simulink model "AME556_Project_Task5_v4"  (R2024b)
settings: Solver=daessc  StartTime=0.0  StopTime=10  FixedStep=0.0005  MaxStep=1e-3  RelTol=1e-2
InitFcn:
  | global params;
  | 
  | % Mass and geometry
  | params.m = 0.25;
  | params.l = 0.22;
  | params.mb = 8;
  | params.a = 0.25;
  | params.b = 0.15;
  | params.g = [0; 9.81; 0];
  | 
  | % Moment of inerita
  | Il_zz = params.m * params.l^2 / 12;
  | Ib_xx = params.mb * params.a^2 / 12;
  | Ib_yy = params.mb * params.b^2 / 12;
  | Ib_zz = params.mb * (params.a^2 + params.b^2) / 12;
  | params.Ib = diag([Ib_xx Ib_yy Ib_zz]);
  | 
  | % Spatial contact force parameters
  | Kp_g = 1e5;
  | Kd_g = 1e3;
  | 
  | % Ground contact positions
  | params.P1 = [0.0197; 0.0022; 0];
  | params.P2 = [0.1838; 0.0041; 0];
  | 
  | % State variables
  | q0 = [0.1; 0.45; 0; -pi/3; pi/2; -pi/6; pi/2]; % Initial states (before landing)
  | params.p_d = [0; 0.5; 0]; % Desired positions (after standing): [x_d; y_d; z_d];
  | params.theta_d = 0; % Desired angle
values from neighbouring files (symbols this model uses):
  dt = 0.04    [AME556_Project_Task5_Setup.m]
  l = 0.5    [AME556_Project_Task5_Setup.m]
  N = 10    [AME556_Project_Task5_Setup.m]
undefined symbols (not defined in the file or in its folder): P1_world0, P2_world0, X, Y, Z
libraries: sm_lib x29, nesl_utility x27
(part 2 of 2)

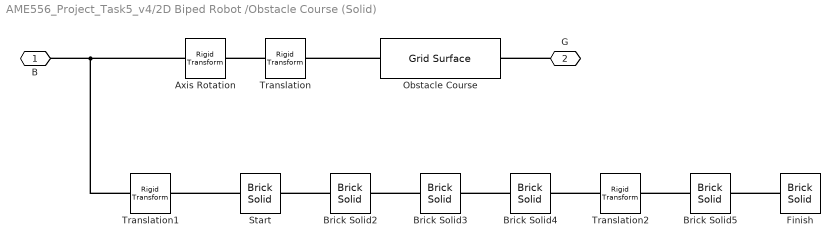
== system AME556_Project_Task5_v4/2D Biped Robot /Obstacle Course (Solid) ==
  Axis Rotation : sm_lib/Frames and Transforms/Rigid Transform  RotationMethod=AlignedAxes  FollAlignAxisA=+X  BaseAlignAxisA=+Z  FollAlignAxisB=+Y  BaseAlignAxisB=+X  RotationStandardAxis=+Z  RotationAngle=0  RotationAngleUnits=deg  RotationArbitraryAxis=[0 0 1]  RotationSequenceAxes=FollowerAxes  RotationSequence=XYX  RotationSequenceAngles=[0 0 0]  RotationSequenceAnglesUnits=deg  RotationMatrix=[1 0 0;0 1 0;0 0 1]  Quaternion=[1 0 0 0]  TranslationMethod=StandardAxis  TranslationCartesianOffset=[0 0 0]  TranslationCartesianOffsetUnits=m  TranslationStandardAxis=-Z  TranslationStandardOffset=0.5  TranslationStandardOffsetUnits=m  TranslationROffset=0  TranslationROffsetUnits=m  TranslationThetaOffset=0  TranslationThetaOffsetUnits=deg  TranslationZOffset=0  TranslationZOffsetUnits=m
  Brick Solid2 : sm_lib/Body Elements/Brick Solid  BrickDimensions=[2 0.4 1]  BrickDimensionsUnits=m  ExportEntireGeometry=off  InertiaType=CalculateFromGeometry  BasedOnType=Density  Density=1000  DensityUnits=kg/m^3  Mass=1  MassUnits=kg  CenterOfMass=[0 0 0]  CenterOfMassUnits=m  MomentsOfInertia=[1 1 1]  MomentsOfInertiaUnits=kg*m^2  ProductsOfInertia=[0 0 0]  ProductsOfInertiaUnits=kg*m^2  GraphicType=FromGeometry  MarkerShape=Sphere  MarkerSize=10  GraphicVisPropType=SimpleVisualProperties  GraphicDiffuseColor=[0.5 0.5 0.5]  GraphicOpacity=1  GraphicSpecularColor=[0.5 0.5 0.5 1.0]  GraphicAmbientColor=[0.15 0.15 0.15 1.0]  GraphicEmissiveColor=[0.0 0.0 0.0 1.0]  GraphicShininess=75  DoExposeReferenceFrame=off  SerializedFrames=<Frames><Frame><Id>Frame1</Id><Value><Name>F1</Name><Origin><Source>GeometricFeature</Source><FeatureName>-x +y curve</FeatureName></Origin><PrimaryAxis><DefinedDirection>+Z</DefinedDirection><Source>ReferenceFrame</Source><SourceDirection>+Z</SourceDirection><FeatureName></FeatureName></PrimaryAxis><SecondaryAxis><DefinedDirection>+X</DefinedDirection><Source>ReferenceFrame</Source><SourceDirection>+X</SourceDirection><FeatureName></FeatureName></SecondaryAxis></Value></Frame><Frame><Id>Frame2</Id><Value><Name>F2</Name><Origin><Source>GeometricFeature</Source><FeatureName>+x -y curve</FeatureName></Origin><PrimaryAxis><DefinedDirection>+Z</DefinedDirection><Source>ReferenceFrame</Source><SourceDirection>+Z</SourceDirection><FeatureName></FeatureName></PrimaryAxis><SecondaryAxis><DefinedDirection>+X</DefinedDirection><Source>ReferenceFrame</Source><SourceDirection>+X</SourceDirection><FeatureName></FeatureName></SecondaryAxis></Value></Frame></Frames>
  Brick Solid3 : sm_lib/Body Elements/Brick Solid  BrickDimensions=[1 0.8 1]  BrickDimensionsUnits=m  ExportEntireGeometry=off  InertiaType=CalculateFromGeometry  BasedOnType=Density  Density=1000  DensityUnits=kg/m^3  Mass=1  MassUnits=kg  CenterOfMass=[0 0 0]  CenterOfMassUnits=m  MomentsOfInertia=[1 1 1]  MomentsOfInertiaUnits=kg*m^2  ProductsOfInertia=[0 0 0]  ProductsOfInertiaUnits=kg*m^2  GraphicType=FromGeometry  MarkerShape=Sphere  MarkerSize=10  GraphicVisPropType=SimpleVisualProperties  GraphicDiffuseColor=[0.5 0.5 0.5]  GraphicOpacity=1  GraphicSpecularColor=[0.5 0.5 0.5 1.0]  GraphicAmbientColor=[0.15 0.15 0.15 1.0]  GraphicEmissiveColor=[0.0 0.0 0.0 1.0]  GraphicShininess=75  DoExposeReferenceFrame=off  SerializedFrames=<Frames><Frame><Id>Frame1</Id><Value><Name>F1</Name><Origin><Source>GeometricFeature</Source><FeatureName>-x -y curve</FeatureName></Origin><PrimaryAxis><DefinedDirection>+Z</DefinedDirection><Source>ReferenceFrame</Source><SourceDirection>+Z</SourceDirection><FeatureName></FeatureName></PrimaryAxis><SecondaryAxis><DefinedDirection>+X</DefinedDirection><Source>ReferenceFrame</Source><SourceDirection>+X</SourceDirection><FeatureName></FeatureName></SecondaryAxis></Value></Frame><Frame><Id>Frame2</Id><Value><Name>F2</Name><Origin><Source>GeometricFeature</Source><FeatureName>+x -y curve</FeatureName></Origin><PrimaryAxis><DefinedDirection>+Z</DefinedDirection><Source>ReferenceFrame</Source><SourceDirection>+Z</SourceDirection><FeatureName></FeatureName></PrimaryAxis><SecondaryAxis><DefinedDirection>+X</DefinedDirection><Source>ReferenceFrame</Source><SourceDirection>+X</SourceDirection><FeatureName></FeatureName></SecondaryAxis></Value></Frame></Frames>
  Brick Solid4 : sm_lib/Body Elements/Brick Solid  BrickDimensions=[2 0.4 1]  BrickDimensionsUnits=m  ExportEntireGeometry=off  InertiaType=CalculateFromGeometry  BasedOnType=Density  Density=1000  DensityUnits=kg/m^3  Mass=1  MassUnits=kg  CenterOfMass=[0 0 0]  CenterOfMassUnits=m  MomentsOfInertia=[1 1 1]  MomentsOfInertiaUnits=kg*m^2  ProductsOfInertia=[0 0 0]  ProductsOfInertiaUnits=kg*m^2  GraphicType=FromGeometry  MarkerShape=Sphere  MarkerSize=10  GraphicVisPropType=SimpleVisualProperties  GraphicDiffuseColor=[0.5 0.5 0.5]  GraphicOpacity=1  GraphicSpecularColor=[0.5 0.5 0.5 1.0]  GraphicAmbientColor=[0.15 0.15 0.15 1.0]  GraphicEmissiveColor=[0.0 0.0 0.0 1.0]  GraphicShininess=75  DoExposeReferenceFrame=off  SerializedFrames=<Frames><Frame><Id>Frame1</Id><Value><Name>F1</Name><Origin><Source>GeometricFeature</Source><FeatureName>-x -y curve</FeatureName></Origin><PrimaryAxis><DefinedDirection>+Z</DefinedDirection><Source>ReferenceFrame</Source><SourceDirection>+Z</SourceDirection><FeatureName></FeatureName></PrimaryAxis><SecondaryAxis><DefinedDirection>+X</DefinedDirection><Source>ReferenceFrame</Source><SourceDirection>+X</SourceDirection><FeatureName></FeatureName></SecondaryAxis></Value></Frame><Frame><Id>Frame2</Id><Value><Name>F2</Name><Origin><Source>GeometricFeature</Source><FeatureName>+x +y curve</FeatureName></Origin><PrimaryAxis><DefinedDirection>+Z</DefinedDirection><Source>ReferenceFrame</Source><SourceDirection>+Z</SourceDirection><FeatureName></FeatureName></PrimaryAxis><SecondaryAxis><DefinedDirection>+X</DefinedDirection><Source>ReferenceFrame</Source><SourceDirection>+X</SourceDirection><FeatureName></FeatureName></SecondaryAxis></Value></Frame></Frames>
  Brick Solid5 : sm_lib/Body Elements/Brick Solid  BrickDimensions=[2 0.4 1]  BrickDimensionsUnits=m  ExportEntireGeometry=off  InertiaType=CalculateFromGeometry  BasedOnType=Density  Density=1000  DensityUnits=kg/m^3  Mass=1  MassUnits=kg  CenterOfMass=[0 0 0]  CenterOfMassUnits=m  MomentsOfInertia=[1 1 1]  MomentsOfInertiaUnits=kg*m^2  ProductsOfInertia=[0 0 0]  ProductsOfInertiaUnits=kg*m^2  GraphicType=FromGeometry  MarkerShape=Sphere  MarkerSize=10  GraphicVisPropType=SimpleVisualProperties  GraphicDiffuseColor=[0.5 0.5 0.5]  GraphicOpacity=1  GraphicSpecularColor=[0.5 0.5 0.5 1.0]  GraphicAmbientColor=[0.15 0.15 0.15 1.0]  GraphicEmissiveColor=[0.0 0.0 0.0 1.0]  GraphicShininess=75  DoExposeReferenceFrame=off  SerializedFrames=<Frames><Frame><Id>Frame1</Id><Value><Name>F1</Name><Origin><Source>GeometricFeature</Source><FeatureName>-x +y curve</FeatureName></Origin><PrimaryAxis><DefinedDirection>+Z</DefinedDirection><Source>ReferenceFrame</Source><SourceDirection>+Z</SourceDirection><FeatureName></FeatureName></PrimaryAxis><SecondaryAxis><DefinedDirection>+X</DefinedDirection><Source>ReferenceFrame</Source><SourceDirection>+X</SourceDirection><FeatureName></FeatureName></SecondaryAxis></Value></Frame><Frame><Id>Frame2</Id><Value><Name>F2</Name><Origin><Source>GeometricFeature</Source><FeatureName>+x +y curve</FeatureName></Origin><PrimaryAxis><DefinedDirection>+Z</DefinedDirection><Source>ReferenceFrame</Source><SourceDirection>+Z</SourceDirection><FeatureName></FeatureName></PrimaryAxis><SecondaryAxis><DefinedDirection>+X</DefinedDirection><Source>ReferenceFrame</Source><SourceDirection>+X</SourceDirection><FeatureName></FeatureName></SecondaryAxis></Value></Frame></Frames>
  Finish : sm_lib/Body Elements/Brick Solid  BrickDimensions=[l 0.4 1]  BrickDimensionsUnits=m  ExportEntireGeometry=off  InertiaType=CalculateFromGeometry  BasedOnType=Density  Density=1000  DensityUnits=kg/m^3  Mass=1  MassUnits=kg  CenterOfMass=[0 0 0]  CenterOfMassUnits=m  MomentsOfInertia=[1 1 1]  MomentsOfInertiaUnits=kg*m^2  ProductsOfInertia=[0 0 0]  ProductsOfInertiaUnits=kg*m^2  GraphicType=FromGeometry  MarkerShape=Sphere  MarkerSize=10  GraphicVisPropType=SimpleVisualProperties  GraphicDiffuseColor=[0 1 0]  GraphicOpacity=1  GraphicSpecularColor=[0.5 0.5 0.5 1.0]  GraphicAmbientColor=[0.15 0.15 0.15 1.0]  GraphicEmissiveColor=[0.0 0.0 0.0 1.0]  GraphicShininess=75  DoExposeReferenceFrame=off  SerializedFrames=<Frames><Frame><Id>Frame1</Id><Value><Name>F1</Name><Origin><Source>GeometricFeature</Source><FeatureName>-x +y curve</FeatureName></Origin><PrimaryAxis><DefinedDirection>+Z</DefinedDirection><Source>ReferenceFrame</Source><SourceDirection>+Z</SourceDirection><FeatureName></FeatureName></PrimaryAxis><SecondaryAxis><DefinedDirection>+X</DefinedDirection><Source>ReferenceFrame</Source><SourceDirection>+X</SourceDirection><FeatureName></FeatureName></SecondaryAxis></Value></Frame></Frames>
  Obstacle Course : sm_lib/Curves and Surfaces/Grid Surface  XGridVector=x_grid  XGridVectorUnits=m  YGridVector=y_grid  YGridVectorUnits=m  ZHeights=z_height  ZHeightsUnits=m  GraphicType=FromGeometry  GraphicVisPropType=SimpleVisualProperties  GraphicDiffuseColor=[1 1 1]  GraphicOpacity=1  GraphicSpecularColor=[0.5 0.5 0.5 1.0]  GraphicAmbientColor=[0.15 0.15 0.15 1.0]  GraphicEmissiveColor=[0.0 0.0 0.0 1.0]  GraphicShininess=75
  Start : sm_lib/Body Elements/Brick Solid  BrickDimensions=[l 0.4 1]  BrickDimensionsUnits=m  ExportEntireGeometry=off  InertiaType=CalculateFromGeometry  BasedOnType=Density  Density=1000  DensityUnits=kg/m^3  Mass=1  MassUnits=kg  CenterOfMass=[0 0 0]  CenterOfMassUnits=m  MomentsOfInertia=[1 1 1]  MomentsOfInertiaUnits=kg*m^2  ProductsOfInertia=[0 0 0]  ProductsOfInertiaUnits=kg*m^2  GraphicType=FromGeometry  MarkerShape=Sphere  MarkerSize=10  GraphicVisPropType=SimpleVisualProperties  GraphicDiffuseColor=[1 0 0]  GraphicOpacity=1  GraphicSpecularColor=[0.5 0.5 0.5 1.0]  GraphicAmbientColor=[0.15 0.15 0.15 1.0]  GraphicEmissiveColor=[0.0 0.0 0.0 1.0]  GraphicShininess=75  DoExposeReferenceFrame=off  SerializedFrames=<Frames><Frame><Id>Frame1</Id><Value><Name>F1</Name><Origin><Source>GeometricFeature</Source><FeatureName>-x +y curve</FeatureName></Origin><PrimaryAxis><DefinedDirection>+Z</DefinedDirection><Source>ReferenceFrame</Source><SourceDirection>+Z</SourceDirection><FeatureName></FeatureName></PrimaryAxis><SecondaryAxis><DefinedDirection>+X</DefinedDirection><Source>ReferenceFrame</Source><SourceDirection>+X</SourceDirection><FeatureName></FeatureName></SecondaryAxis></Value></Frame><Frame><Id>Frame2</Id><Value><Name>F2</Name><Origin><Source>GeometricFeature</Source><FeatureName>+x +y curve</FeatureName></Origin><PrimaryAxis><DefinedDirection>+Z</DefinedDirection><Source>ReferenceFrame</Source><SourceDirection>+Z</SourceDirection><FeatureName></FeatureName></PrimaryAxis><SecondaryAxis><DefinedDirection>+X</DefinedDirection><Source>ReferenceFrame</Source><SourceDirection>+X</SourceDirection><FeatureName></FeatureName></SecondaryAxis></Value></Frame></Frames>
  Translation : sm_lib/Frames and Transforms/Rigid Transform  RotationMethod=None  FollAlignAxisA=+X  BaseAlignAxisA=+Z  FollAlignAxisB=+Y  BaseAlignAxisB=+X  RotationStandardAxis=+Z  RotationAngle=0  RotationAngleUnits=deg  RotationArbitraryAxis=[0 0 1]  RotationSequenceAxes=FollowerAxes  RotationSequence=XYX  RotationSequenceAngles=[0 0 0]  RotationSequenceAnglesUnits=deg  RotationMatrix=[1 0 0;0 1 0;0 0 1]  Quaternion=[1 0 0 0]  TranslationMethod=StandardAxis  TranslationCartesianOffset=[0 0 0]  TranslationCartesianOffsetUnits=m  TranslationStandardAxis=-Y  TranslationStandardOffset=l  TranslationStandardOffsetUnits=m  TranslationROffset=0  TranslationROffsetUnits=m  TranslationThetaOffset=0  TranslationThetaOffsetUnits=deg  TranslationZOffset=0  TranslationZOffsetUnits=m
  Translation1 : sm_lib/Frames and Transforms/Rigid Transform  RotationMethod=None  FollAlignAxisA=+X  BaseAlignAxisA=+Z  FollAlignAxisB=+Y  BaseAlignAxisB=+X  RotationStandardAxis=+Z  RotationAngle=0  RotationAngleUnits=deg  RotationArbitraryAxis=[0 0 1]  RotationSequenceAxes=FollowerAxes  RotationSequence=XYX  RotationSequenceAngles=[0 0 0]  RotationSequenceAnglesUnits=deg  RotationMatrix=[1 0 0;0 1 0;0 0 1]  Quaternion=[1 0 0 0]  TranslationMethod=StandardAxis  TranslationCartesianOffset=[0 0 0]  TranslationCartesianOffsetUnits=m  TranslationStandardAxis=-X  TranslationStandardOffset=l  TranslationStandardOffsetUnits=m  TranslationROffset=0  TranslationROffsetUnits=m  TranslationThetaOffset=0  TranslationThetaOffsetUnits=deg  TranslationZOffset=0  TranslationZOffsetUnits=m
  Translation2 : sm_lib/Frames and Transforms/Rigid Transform  RotationMethod=None  FollAlignAxisA=+X  BaseAlignAxisA=+Z  FollAlignAxisB=+Y  BaseAlignAxisB=+X  RotationStandardAxis=+Z  RotationAngle=0  RotationAngleUnits=deg  RotationArbitraryAxis=[0 0 1]  RotationSequenceAxes=FollowerAxes  RotationSequence=XYX  RotationSequenceAngles=[0 0 0]  RotationSequenceAnglesUnits=deg  RotationMatrix=[1 0 0;0 1 0;0 0 1]  Quaternion=[1 0 0 0]  TranslationMethod=StandardAxis  TranslationCartesianOffset=[0 0 0]  TranslationCartesianOffsetUnits=m  TranslationStandardAxis=+X  TranslationStandardOffset=0.4  TranslationStandardOffsetUnits=m  TranslationROffset=0  TranslationROffsetUnits=m  TranslationThetaOffset=0  TranslationThetaOffsetUnits=deg  TranslationZOffset=0  TranslationZOffsetUnits=m
  Β : PMIOPort  Side=Left
  G : PMIOPort  Port=2  Side=Right
  connections:
  Translation1/LConn1 -- Β/RConn1 -- Axis Rotation/LConn1
  Brick Solid4/LConn1 -- Brick Solid3/RConn1
  Brick Solid2/LConn1 -- Start/RConn1
  Translation2/LConn1 -- Brick Solid4/RConn1
  Finish/LConn1 -- Brick Solid5/RConn1
  Brick Solid5/LConn1 -- Translation2/RConn1
  Brick Solid3/LConn1 -- Brick Solid2/RConn1
  Start/LConn1 -- Translation1/RConn1
  Obstacle Course/LConn1 -- Translation/RConn1
  Translation/LConn1 -- Axis Rotation/RConn1
  G/RConn1 -- Obstacle Course/RConn1

== matlab function AME556_Project_Task5_v4/MATLAB Function ==
  data: tau_unsaturated input; tau_saturated output; saturateSwitch input
function tau_saturated = tau_saturation(tau_unsaturated, saturateSwitch)
    if saturateSwitch == 1
        tau_limits = [30, 60, 30, 60];
    
        tau_saturated = tau_unsaturated;
    
        for i = 1:length(tau_unsaturated)
            if tau_unsaturated(i) > tau_limits(i)
                tau_saturated(i) = tau_limits(i);
                warning('Tau %d (%.2f) is saturated to %d', i, tau_unsaturated(i), tau_limits(i));
            elseif tau_unsaturated(i) < -tau_limits(i)
                tau_saturated(i) = -tau_limits(i);
                warning('Tau %d (%.2f) is saturated to -%d', i, tau_unsaturated(i), tau_limits(i));
            end
        end
    else
        tau_saturated = tau_unsaturated;
    end
end

== matlab function AME556_Project_Task5_v4/Controller/Condensed MPC Controller ==
  settings: updateMethod=DISCRETE
  data: p input; theta input; dp input; dtheta input; qs input; tau output; P1 input; P2 input; dP1 input; dP2 input; N input; dt input; t input
%% Function: Low Level Control

function tau = lowLevelControl(p, theta, dp, dtheta, qs, P1, P2, dP1, dP2, N, dt, t)

% 正常情况下我们就正常摆腿
if p(1)<=1.7
    gaitType = "walk"; % Walk from start

elseif p(1)>1.7 && p(1)<=2.1
    gaitType = "hop_stand"; % Ready to jump

    if P1(2)>0.05 && P2(2)>0.05 % Flight
        gaitType = "hop_flight"; 
    end
    
elseif p(1)>2.1 && p(1)<=3
    gaitType = "walk_on_obstacle"; % Walk on higher ground

elseif p(1)>3 && p(1)<=4
    gaitType = "walk"; % 

elseif p(1)>4 && p(1)<=4.9
    gaitType = "walk2"; % 回到平地走

elseif p(1)>4.9 && p(1)<=5.4
    gaitType = "gap"; 
    
    if P1(1)>5.4
        gaitType = "stand"; 
    end
    if P2(1)>5.0
        gaitType = "stand2";
    end

else
    gaitType = "walk2";
end

% disp(gaitType)

con = gaitSchedule(N, dt, t, gaitType);
F = condensed_mpc_controller(p, theta, dp, dtheta, P1, P2, N, dt, t, con, gaitType);
J = jacobianFcn(theta, qs);

tau = zeros(4, 1);
if con(1, 1) && con(2, 1)
    tau = -J' * F;
elseif con(1, 1) && ~con(2, 1)
    F_swing = swingLegControl(p, dp, P2, dP2, N, dt, t, gaitType);
    F_new = [F(1: 2); -F_swing];
    tau = -J' * F_new;
elseif con(2, 1) && ~con(1, 1)
    F_swing = swingLegControl(p, dp, P1, dP1, N, dt, t, gaitType);
    F_new = [-F_swing; F(3: 4)];
    tau = -J' * F_new;
else
    F_swing1 = swingLegControl(p, dp, P1, dP1, N, dt, t, gaitType);
    F_swing2 = swingLegControl(p, dp, P2, dP2, N, dt, t, gaitType);
    F_new = [-F_swing1; -F_swing2];
    tau = -J' * F_new;    
end

end

%% Function: Condensed MPC Controller

function F = condensed_mpc_controller(p, theta, dp, dtheta, P1, P2, N, dt, t, con, gaitType)

% Parameters
mt = 8;
a = 0.25;
b = 0.15;
g = [0; 9.81; 0];
Ib_zz = mt * (a^2 + b^2) / 12;

numStates = 7;
numCtrls = 4;
Q = diag([200 200 800 30 10 10 0]);
R = 0.0001*eye(numCtrls);

% q = [x; y; z; R1; dx; dy; dz; wbx; wby; wbz];
% X = [x; y; theta; dx; dy; dtheta; g];
X = zeros(numStates, 1);
X(1: 2) = p;
X(3) = theta;
X(4: 5) = dp;
X(6) = dtheta;
X(7) = g(2);

% Desired states
switch gaitType
    case "walk"
        X_d = [0.5*t; 0.40; 0; 0.5; 0; 0; g(2)];

    case "jump_up"
        X_d = [0.5*t; 0.80; 0; dp(1); 3; 0; g(2)]; 

    case "fly_up"
        % fly的时候其实都是F_swing，不计算mpc，直接return
        F = zeros(4,1);
        return;

    case "walk_on_obstacle"
        X_d = [p(1); 0.80; 0; 0; 0; 0; g(2)];
    
    case "walk2"
        X_d = [0.8*t; 0.40; 0; 0.8; 0; 0; g(2)];

    case "gap"
        X_d = [5.40; 0.40; 0; dp(1); 0; 0; g(2)];

    case "stand"
        X_d = [5.40; 0.40; 0; dp(1); 0; 0; g(2)];
    case "stand2"
        X_d = [5.40; 0.40; 0; dp(1); 0; 0; g(2)];       

    otherwise
        error("unknown gait type");
end


% Reference Trajectory
X_ref = getReferenceTrajectory(dt, N, p, theta, dp, dtheta, X_d);
y = reshape(X_ref, [numStates*N 1]);

r1 = P1 - p;
r2 = P2 - p;

% Linearized system (A, B)
A = [zeros(3)   eye(3)    zeros(3,1);
     zeros(3, numStates-1) [0; -1; 0];
     zeros(1, numStates)];

B = [zeros(3, numCtrls);
     eye(2)/mt eye(2)/mt;
     -r1(2)/Ib_zz r1(1)/Ib_zz -r2(2)/Ib_zz r2(1)/Ib_zz;
     zeros(1, numCtrls)];

% Discrete-time system matrices (Ak, Bk)
Ak = A * dt + eye(size(A, 1));
Bk = B * dt;

% Aqp
Aqp = [];
for i = 1: N
    Aqp = [Aqp; mpower(Ak, i)];
end

% bqp
Bqp = repmat(zeros(size(Bk)), N, N);
for i = 0: N-1
    element = mpower(Ak, i) * Bk;
    Bqp = Bqp + kron(diag(ones(1, N - i), -i), element);
end

% Condensation
L = kron(eye(N), Q);
K = kron(eye(N), R);

% Optimization weights (H, f)
H = 2*(Bqp'*L*Bqp + K);
f = 2*Bqp'*L*(Aqp*X - y);

% Inequality constraints (A_ineq, b_ineq)
Aineq_mu = kron(eye(2), [1 -0.7; -1 -0.7]);
Aineq_mu_N = kron(eye(N), Aineq_mu);
Aineq_F = kron(eye(2), [0 1; 0 -1]);
Aineq_F_N = kron(eye(N), Aineq_F);
Aineq = [Aineq_mu_N; Aineq_F_N];

bineq_mu = repmat([0; 0; 0; 0], N, 1);
bineq_f = [];
for i = 1: N
    bineq_f = [bineq_f; [250; -10]*con(1, i); [250; -10]*con(2, i)];
end
bineq = [bineq_mu; bineq_f];

% Initial guess
u0 = zeros(length(f), 1);

% Quadratic programming
options = optimoptions('quadprog', 'Algorithm', 'active-set', 'Display', 'off');
u_mpc = quadprog(H, f, Aineq, bineq, [], [], [], [], u0, options);

% Force inputs
F = u_mpc(1: numCtrls);

end


%% Function: Get Reference Geometry

function X_ref = getReferenceTrajectory(dt, N, p, theta, dp, dtheta, X_d)

X = [p; theta; dp; dtheta; 9.81];
X_ref = repmat(X, 1, N);

for i = 1: 3
    for k = 2: N
        if X_d(i + 3) ~= 0
            X_ref(i, k) = X(i) + X_d(i+3)*((k-1)*dt);
        else
            X_ref(i, k) = X_d(i);
        end
    end
end

end

%% Function: Swing Leg Control

function F_swing = swingLegControl(p, dp, P, dP, N, dt, t, gaitType)

Kp = diag([200 300]);
Kd = eye(2)*5;

del_t = N*dt/2;
ts = rem(t, del_t);

switch gaitType
    case "walk"
        % 正常摆腿逻辑
        swingHeight = 0.1; % 正常摆腿高度
        Px_d = p(1) + (1/2)*del_t*dp(1);
        Py_d = swingHeight * sin(pi*ts/del_t);
    
    case "hop_stand"
        % jump的时候其实双脚落地不会有F_swing，不计算F_swing，直接返回
        F_swing = zeros(2,1);
        return;

    case "hop_fligt"
        % 试图抬高双脚
        swingHeight = 0.2;
        Px_d = p(1) + (1/2)*del_t*dp(1);
        %Py_d = (1/2)*del_t*dp(2) + 2*(sin(pi*ts/del_t))^(1/3)*swingHeight;
        Py_d = 0.5;

    case "walk_on_obstacle"
        % 正常摆腿逻辑
        swingHeight = 0.1; % 正常摆腿高度
        Px_d = p(1) + (1/2)*del_t*dp(1);
        Py_d = (swingHeight+0.4) * sin(pi*ts/del_t);

    case "walk2"
        % 正常摆腿逻辑
        swingHeight = 0.1; % 正常摆腿高度
        Px_d = p(1) + (1/2)*del_t*dp(1);
        Py_d = swingHeight * sin(pi*ts/del_t);

    case "gap"
        % 试图单腿迈过沟
        swingHeight = 0.1; 
        Px_d = 5.8;
        Py_d = swingHeight * sin(pi*ts/del_t);
    
    case "stand"
        % stand的时候其实双脚落地不会有F_swing，不计算F_swing，直接返回
        F_swing = zeros(2,1);
        return;

    case "stand2"
        % stand的时候其实双脚落地不会有F_swing，不计算F_swing，直接返回
        swingHeight = 0.1; 
        Px_d = 5.8;
        Py_d = swingHeight * sin(pi*ts/del_t);

    otherwise
        error("unknown gait type");
end

F_swing = Kp*([Px_d; Py_d] - P) + Kd*(0 - dP);

end

%% Function: Jacobian Function
% Convert contact forces to joint torques

function J = jacobianFcn(theta, qs)

l = 0.22;

q1 = qs(1); q2 = qs(2); q3 = qs(3); q4 = qs(4);

J = [l*cos(q1 + q2 + theta) + l*cos(q1 + theta), l*cos(q1 + q2 + theta),                                          0,                      0;
     l*sin(q1 + q2 + theta) + l*sin(q1 + theta), l*sin(q1 + q2 + theta),                                          0,                      0;
                                              0,                      0, l*cos(q3 + q4 + theta) + l*cos(q3 + theta), l*cos(q3 + q4 + theta);
                                              0,                      0, l*sin(q3 + q4 + theta) + l*sin(q3 + theta), l*sin(q3 + q4 + theta)];

end

%% Function: Gait Schedule
% Generate gait schedule based on walking phase

function sigma = gaitSchedule(N, dt, t, gaitType)
    % gaitType: 步态类型，字符串形式（例如 "walk", "jump", "aerial"）

    % 初始化步态矩阵
    sigma_l0 = []; % 左腿步态
    sigma_r0 = []; % 右腿步态

    % 根据步态类型切换逻辑
    switch gaitType
        case "walk"
            sigma_l0 = [ones(1, N/2) zeros(1, N/2)]; 
            sigma_r0 = [zeros(1, N/2) ones(1, N/2)]; 

        case "hop_stand"
            sigma = ones(2, N); % 两腿均站在地面上
            return;

        case "hop_flight"
            sigma = zeros(2, N); % 两腿均腾空
            return;

        case "walk_on_obstacle"
            sigma_l0 = [ones(1, N/2) zeros(1, N/2)]; 
            sigma_r0 = [zeros(1, N/2) ones(1, N/2)]; 

        case "walk2"
            sigma_l0 = [ones(1, N/2) zeros(1, N/2)]; 
            sigma_r0 = [zeros(1, N/2) ones(1, N/2)]; 

        case "gap"
            sigma_l0 = [ones(1, N/2) zeros(1, N/2)]; 
            sigma_r0 = [zeros(1, N/2) ones(1, N/2)]; 

        case "stand"
            sigma = ones(2, N); % 两腿均站在地面上
            return;

        case "stand2"
            sigma_l0 = [ones(1, N)]; 
            sigma_r0 = [zeros(1, N)]; 

        otherwise
            error("unknown gait type");
    end

    % 根据当前时间步调整步态
    phase = floor(t/dt); % 当前周期阶段
    k = rem(phase, N);   % 当前周期位置

    if k ~= 0
        % 调整步态使其与当前周期对齐
        sigma_l = [sigma_l0(k+1: N) sigma_l0(1: k)];
        sigma_r = [sigma_r0(k+1: N) sigma_r0(1: k)];
    else
        % 当前周期不需要调整
        sigma_l = sigma_l0;
        sigma_r = sigma_r0;
    end

    % 合并步态矩阵
    sigma = [sigma_l; sigma_r];
end
